simulink model "PitchDamper"  (R2021b)
settings: Solver=VariableStepAuto  StartTime=0.0  StopTime=100  RelTol=1e-3
values from neighbouring files (symbols this model uses):
  max_dev_elevator = 25 - trim_control_lo(1)    [Glideslope.m]
  min_dev_elevator = -25 - trim_control_lo(1)    [Glideslope.m]
libraries: cstblocks x1
settings Model: Creator=ddefu  LastModifiedBy=ddefu

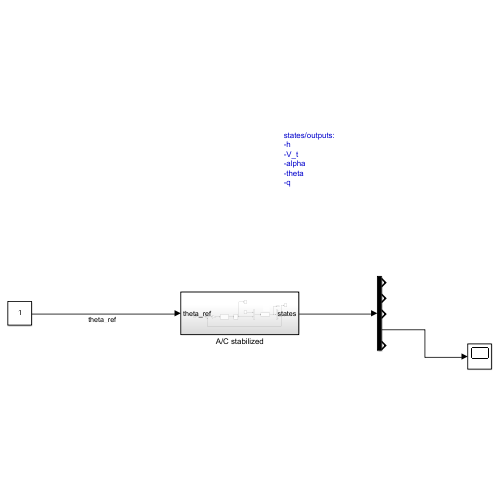
[thumbnail: Simulink's stored preview of the top-level diagram]
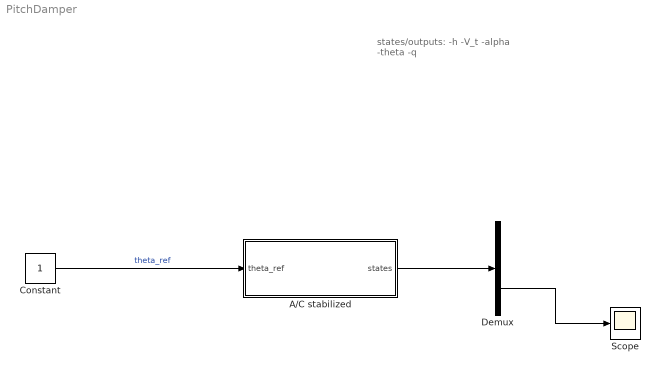
== system PitchDamper ==
  note: states/outputs:
      | -h
      | -V_t
      | -alpha
      | -theta
      | -q
  A/C stabilized : Subsystem
  Constant : Constant
  Demux : Demux  Outputs=5
  Scope : Scope
  wires:
  Constant/1 -> A/C stabilized/1(theta_ref)  "theta_ref"
  A/C stabilized/1(states) -> Demux/1
  Demux/4 -> Scope/1

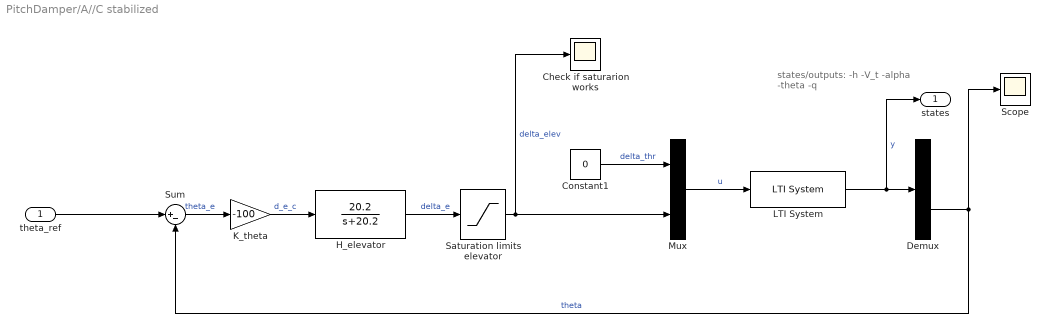
== system PitchDamper/A//C stabilized ==
  note: states/outputs:
      | -h
      | -V_t
      | -alpha
      | -theta
      | -q
  theta_ref : Inport
  Check if saturarion works : Scope
  Constant1 : Constant  Value=0
  Demux : Demux  Outputs=5
  H_elevator : TransferFcn  Numerator=[20.2]  Denominator=[1 20.2]
  K_theta : Gain  Gain=-100
  LTI System : cstblocks/LTI System  sys=sys_reduced  IC=[0;0;0;0;0]
  Mux : Mux  Inputs=2
  Saturation limits elevator : Saturate  UpperLimit=max_dev_elevator  LowerLimit=min_dev_elevator
  Scope : Scope
  Sum : Sum  Inputs=|+-
  states : Outport
  wires:
  LTI System/1 -> Demux/1, states/1  "y"
  theta_ref/1 -> Sum/1
  K_theta/1 -> H_elevator/1  "d_e_c"
  Constant1/1 -> Mux/1  "delta_thr"
  Mux/1 -> LTI System/1  "u"
  Demux/4 -> Scope/1, Sum/2  "theta"
  Sum/1 -> K_theta/1  "theta_e"
  H_elevator/1 -> Saturation limits elevator/1  "delta_e"
  Saturation limits elevator/1 -> Check if saturarion works/1, Mux/2  "delta_elev"
